simulink library "calc_angle_between_vectors"  (R2020a)
settings: Solver=VariableStepAuto  StartTime=0.0  StopTime=10.0  RelTol=1e-3
libraries: vrlib x2
settings Model: Creator=Ayaz  LastModifiedBy=Ayaz

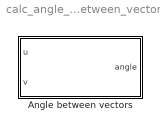
== system calc_angle_between_vectors ==
  Angle between vectors : Subsystem

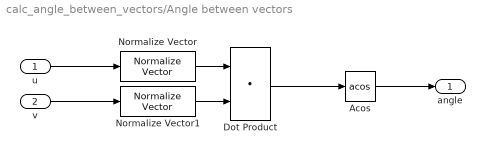
== system calc_angle_between_vectors/Angle between vectors ==
  u : Inport
  v : Inport  Port=2
  Acos : Trigonometry  Operator=acos
  Dot Product : DotProduct  InputSameDT=on  OutDataTypeStr=Inherit: Inherit via internal rule
  Normalize Vector : vrlib/Utilities/Normalize Vector  maxzero=0
  Normalize Vector1 : vrlib/Utilities/Normalize Vector  maxzero=0
  angle : Outport
  wires:
  v/1 -> Normalize Vector1/1
  u/1 -> Normalize Vector/1
  Dot Product/1 -> Acos/1
  Acos/1 -> angle/1
  Normalize Vector/1 -> Dot Product/1
  Normalize Vector1/1 -> Dot Product/2
